simulink model "hil_tuning"  (R2018a)
settings: Solver=FixedStepAuto  StartTime=0.0  StopTime=inf  FixedStep=0.001  RelTol=1e-3  EnableMultiTasking=on
undefined symbols (not defined in the file or in its folder): d
libraries: simulink x12, xpcrtudplib x3, xpcseriallib x2
settings Model: SimulationMode=external  Creator=KLETech  LastModifiedBy=KLETech
settings SolverCC: ConcurrentTasks=on  AutoInsertRateTranBlk=on
settings DataIOCC: SaveFormat=StructureWithTime
settings OptimizationCC: BlockReduction=off  OptimizeBlockIOStorage=off  BufferReuse=off  GlobalBufferReuse=off  ExpressionFolding=off  LocalBlockOutputs=off  OptimizeDataStoreBuffers=off  BusAssignmentInplaceUpdate=off
settings HardwareCC: ProdBitPerPointer=32  ProdBitPerSizeT=32  ProdBitPerPtrDiffT=32  ProdLargestAtomicFloat=None  ProdWordSize=32  ProdLongLongMode=on  ProdHWDeviceType=Generic->32-bit x86 compatible
settings RTWCC: SystemTargetFile=slrt.tlc  TemplateMakefile=slrt_default_tmf  Description=Simulink Real-Time  CodeExecutionProfiling=on  RTWCompilerOptimization=on
settings SimulinkRealTimeCC: SupportVariableSizeSignals=on  RL32LogTETModifier=off  xPCConcurrentTasks=on

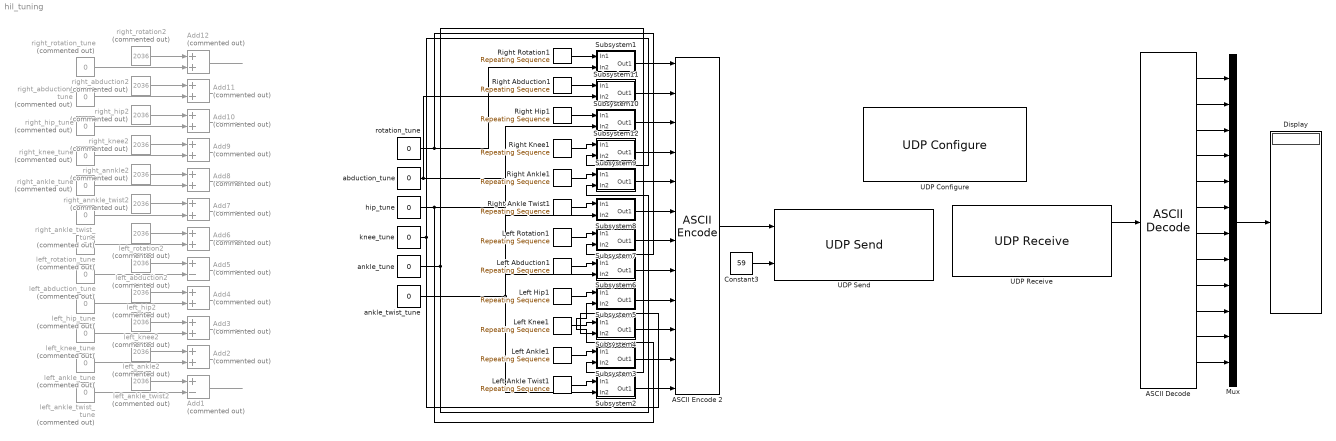
== system hil_tuning ==
  "ASCII Decode " : xpcseriallib/ASCII Decode   format=%d,%d,%d,%d,%d,%d,%d,%d,%d,%d,%d,%d  nvars=12  vartypes={ 'uint32' }
      settings: SourceProductName=Simulink Real-Time  SourceProductBaseCode=XP
  ASCII Encode 2 : xpcseriallib/ASCII Encode   format=%d,%d,%d,%d,%d,%d,%d,%d,%d,%d,%d,%d  nvars=12  maxlength=128  vartypes={ 'uint32' }
      settings: SourceProductName=Simulink Real-Time  SourceProductBaseCode=XP
  Add1 : Sum  Commented=on  Inputs=+-  OutDataTypeStr=uint32
  Add{2..4,6..12} (10 alike) : Sum  Commented=on  OutDataTypeStr=uint32
  Add5 : Sum  Commented=on  Inputs=+-  OutDataTypeStr=uint32
  Constant3 : Constant  Value=59
  Display : Display
  Left Abduction1 : simulink/Sources/Repeating Sequence  rep_seq_t=time  rep_seq_y=left_abduction
  Left Ankle Twist1 : simulink/Sources/Repeating Sequence  rep_seq_t=time  rep_seq_y=left_knee_twist
  Left Ankle1 : simulink/Sources/Repeating Sequence  rep_seq_t=time  rep_seq_y=left_ankle
  Left Hip1 : simulink/Sources/Repeating Sequence  rep_seq_t=time  rep_seq_y=left_hip
  Left Knee1 : simulink/Sources/Repeating Sequence  rep_seq_t=time  rep_seq_y=left_knee
  Left Rotation1 : simulink/Sources/Repeating Sequence  rep_seq_t=time  rep_seq_y=left_rotation
  Mux : Mux  Inputs=12
  Right Abduction1 : simulink/Sources/Repeating Sequence  rep_seq_t=time  rep_seq_y=right_abduction
  Right Ankle Twist1 : simulink/Sources/Repeating Sequence  rep_seq_t=time  rep_seq_y=right_knee_twist
  Right Ankle1 : simulink/Sources/Repeating Sequence  rep_seq_t=time  rep_seq_y=right_ankle
  Right Hip1 : simulink/Sources/Repeating Sequence  rep_seq_t=time  rep_seq_y=right_hip
  Right Knee1 : simulink/Sources/Repeating Sequence  rep_seq_t=time  rep_seq_y=right_knee
  Right Rotation1 : simulink/Sources/Repeating Sequence  rep_seq_t=time  rep_seq_y=right_rotation
  Subsystem1 : Subsystem
  Subsystem10 : Subsystem
  Subsystem11 : Subsystem
  Subsystem12 : Subsystem
  Subsystem2 : Subsystem
  Subsystem3 : Subsystem
  Subsystem4 : Subsystem
  Subsystem5 : Subsystem
  Subsystem6 : Subsystem
  Subsystem7 : Subsystem
  Subsystem8 : Subsystem
  Subsystem9 : Subsystem
  UDP Configure : xpcrtudplib/UDP Configure  Priority=-1  IpAddress=192.168.7.3  SubnetMask=255.0.0.0  Gateway=0.0.0.0  PciBus=[2]  PciSlot=[0]  PciFunction=0  ID=1  tune=0  enableMulticast=on  MulticastIpAddress={}  MulticastMask={}
      settings: SourceProductName=Simulink Real-Time  SourceProductBaseCode=XP
  UDP Receive : xpcrtudplib/UDP Receive  ipAddressVal=192.168.7.3  localPort=1234  rcvWidth=128  rcvFmAny=off  fmAddress=192.168.2.101  rcvMulticast=off  multicastAddress=[]  maxUDPQueue=8  sampleTime=-1
      settings: SourceProductName=Simulink Real-Time
  UDP Send : xpcrtudplib/UDP Send  ipAddressVal=192.168.7.3  localPort=25001  toAddress=192.168.2.101  toPort=8001  sampleTime=-1
      settings: SourceProductName=Simulink Real-Time  SourceProductBaseCode=XP
  abduction_tune : Constant  Value=0
  ankle_tune : Constant  Value=0
  ankle_twist_tune : Constant  Value=0
  hip_tune : Constant  Value=0
  knee_tune : Constant  Value=0
  "left_abduction2 " : Constant  Commented=on  Value=2036  OutDataTypeStr=uint32
  left_abduction_tune : Constant  Commented=on  Value=0  OutDataTypeStr=int32
  left_ankle2 : Constant  Commented=on  Value=2036  OutDataTypeStr=uint32
  left_ankle_tune : Constant  Commented=on  Value=0  OutDataTypeStr=int32
  "left_ankle_twist2 " : Constant  Commented=on  Value=2036  OutDataTypeStr=uint32
  left_ankle_twist_tune : Constant  Commented=on  Value=0  OutDataTypeStr=int32
  "left_hip2 " : Constant  Commented=on  Value=2036  OutDataTypeStr=uint32
  left_hip_tune : Constant  Commented=on  Value=0  OutDataTypeStr=int32
  left_knee2 : Constant  Commented=on  Value=2036  OutDataTypeStr=uint32
  left_knee_tune : Constant  Commented=on  Value=0  OutDataTypeStr=int32
  "left_rotation2 " : Constant  Commented=on  Value=2036  OutDataTypeStr=uint32
  left_rotation_tune : Constant  Commented=on  Value=0  OutDataTypeStr=int32
  "right_abduction2 " : Constant  Commented=on  Value=2036  OutDataTypeStr=uint32
  right_abduction_tune : Constant  Commented=on  Value=0  OutDataTypeStr=int32
  right_ankle_tune : Constant  Commented=on  Value=0  OutDataTypeStr=int32
  right_ankle_twist_tune : Constant  Commented=on  Value=0  OutDataTypeStr=int32
  right_annkle2 : Constant  Commented=on  Value=2036  OutDataTypeStr=uint32
  "right_annkle_twist2 " : Constant  Commented=on  Value=2036  OutDataTypeStr=uint32
  "right_hip2 " : Constant  Commented=on  Value=2036  OutDataTypeStr=uint32
  right_hip_tune : Constant  Commented=on  Value=0  OutDataTypeStr=int32
  right_knee2 : Constant  Commented=on  Value=2036  OutDataTypeStr=uint32
  right_knee_tune : Constant  Commented=on  Value=0  OutDataTypeStr=int32
  right_rotation2 : Constant  Commented=on  Value=2036  OutDataTypeStr=uint32
  right_rotation_tune : Constant  Commented=on  Value=0  OutDataTypeStr=int32
  rotation_tune : Constant  Value=0
  wires:
  ASCII Encode 2/1 -> UDP Send/1
  Constant3/1 -> UDP Send/2
  UDP Receive/1 -> "ASCII Decode "/1
  "ASCII Decode "/1 -> Mux/1
  "ASCII Decode "/2 -> Mux/2
  "ASCII Decode "/3 -> Mux/3
  "ASCII Decode "/4 -> Mux/4
  "ASCII Decode "/5 -> Mux/5
  "ASCII Decode "/6 -> Mux/6
  "ASCII Decode "/7 -> Mux/7
  "ASCII Decode "/8 -> Mux/8
  "ASCII Decode "/9 -> Mux/9
  "ASCII Decode "/10 -> Mux/10
  "ASCII Decode "/11 -> Mux/11
  "ASCII Decode "/12 -> Mux/12
  Mux/1 -> Display/1
  Subsystem7/1(Out1) -> ASCII Encode 2/7
  Subsystem1/1(Out1) -> ASCII Encode 2/1
  Subsystem10/1(Out1) -> ASCII Encode 2/3
  Subsystem12/1(Out1) -> ASCII Encode 2/4
  Subsystem9/1(Out1) -> ASCII Encode 2/5
  Subsystem5/1(Out1) -> ASCII Encode 2/9
  Subsystem3/1(Out1) -> ASCII Encode 2/11
  Subsystem11/1(Out1) -> ASCII Encode 2/2
  Subsystem4/1(Out1) -> ASCII Encode 2/10
  Right Abduction1/1 -> Subsystem11/1(In1)
  Right Rotation1/1 -> Subsystem1/1(In1)
  Left Rotation1/1 -> Subsystem7/1(In1)
  Subsystem8/1(Out1) -> ASCII Encode 2/6
  Subsystem6/1(Out1) -> ASCII Encode 2/8
  Subsystem2/1(Out1) -> ASCII Encode 2/12
  Left Ankle Twist1/1 -> Subsystem2/1(In1)
  Left Ankle1/1 -> Subsystem3/1(In1)
  Right Ankle Twist1/1 -> Subsystem8/1(In1)
  Left Hip1/1 -> Subsystem5/1(In1)
  Left Knee1/1 -> Subsystem4/1(In1)
  Right Ankle1/1 -> Subsystem9/1(In1)
  Right Knee1/1 -> Subsystem12/1(In1)
  Right Hip1/1 -> Subsystem10/1(In1)
  Left Abduction1/1 -> Subsystem6/1(In1)
  "left_ankle_twist2 "/1 -> Add1/1
  "right_abduction2 "/1 -> Add11/1
  "right_hip2 "/1 -> Add10/1
  left_knee2/1 -> Add3/1
  right_knee2/1 -> Add9/1
  "left_abduction2 "/1 -> Add5/1
  left_ankle2/1 -> Add2/1
  "left_rotation2 "/1 -> Add6/1
  right_rotation2/1 -> Add12/1
  left_ankle_tune/1 -> Add2/2
  right_knee_tune/1 -> Add9/2
  left_rotation_tune/1 -> Add6/2
  right_hip_tune/1 -> Add10/2
  left_abduction_tune/1 -> Add5/2
  right_abduction_tune/1 -> Add11/2
  right_ankle_tune/1 -> Add8/2
  left_knee_tune/1 -> Add3/2
  right_ankle_twist_tune/1 -> Add7/2
  left_hip_tune/1 -> Add4/2
  right_rotation_tune/1 -> Add12/2
  Add6/1 -> ?
  right_annkle2/1 -> Add8/1
  Add10/1 -> ?
  Add12/1 -> ?
  "left_hip2 "/1 -> Add4/1
  Add1/1 -> ?
  Add4/1 -> ?
  Add2/1 -> ?
  Add8/1 -> ?
  Add3/1 -> ?
  "right_annkle_twist2 "/1 -> Add7/1
  Add11/1 -> ?
  Add9/1 -> ?
  Add7/1 -> ?
  Add5/1 -> ?
  left_ankle_twist_tune/1 -> Add1/2
  ankle_twist_tune/1 -> Subsystem8/2(In2), Subsystem2/2(In2)
  ankle_tune/1 -> Subsystem9/2(In2), Subsystem3/2(In2)
  knee_tune/1 -> Subsystem12/2(In2), Subsystem4/2(In2)
  hip_tune/1 -> Subsystem10/2(In2), Subsystem5/2(In2)
  abduction_tune/1 -> Subsystem11/2(In2), Subsystem6/2(In2)
  rotation_tune/1 -> Subsystem7/2(In2), Subsystem1/2(In2)

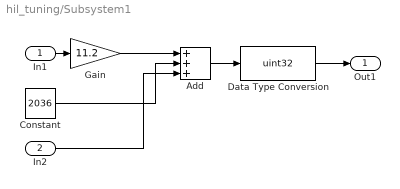
== system hil_tuning/Subsystem1 ==
  In1 : Inport
  In2 : Inport  Port=2
  Add : Sum  Inputs=+++
  Constant : Constant  Value=2036
  Data Type Conversion : DataTypeConversion  OutDataTypeStr=uint32
  Gain : Gain  Gain=11.2
  Out1 : Outport
  wires:
  Add/1 -> Data Type Conversion/1
  Gain/1 -> Add/1
  Constant/1 -> Add/2
  In1/1 -> Gain/1
  Data Type Conversion/1 -> Out1/1
  In2/1 -> Add/3

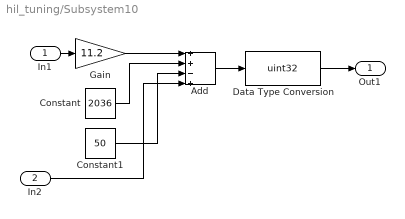
== system hil_tuning/Subsystem10 ==
  In1 : Inport
  In2 : Inport  Port=2
  Add : Sum  Inputs=++-+
  Constant : Constant  Value=2036
  Constant1 : Constant  Value=50
  Data Type Conversion : DataTypeConversion  OutDataTypeStr=uint32
  Gain : Gain  Gain=11.2
  Out1 : Outport
  wires:
  Add/1 -> Data Type Conversion/1
  Gain/1 -> Add/1
  Constant/1 -> Add/2
  In1/1 -> Gain/1
  Data Type Conversion/1 -> Out1/1
  Constant1/1 -> Add/3
  In2/1 -> Add/4

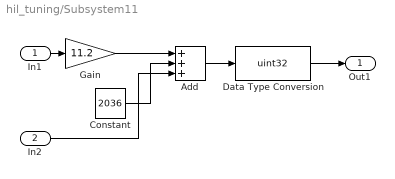
== system hil_tuning/Subsystem11 ==
  In1 : Inport
  In2 : Inport  Port=2
  Add : Sum  Inputs=+++
  Constant : Constant  Value=2036
  Data Type Conversion : DataTypeConversion  OutDataTypeStr=uint32
  Gain : Gain  Gain=11.2
  Out1 : Outport
  wires:
  Add/1 -> Data Type Conversion/1
  Gain/1 -> Add/1
  Constant/1 -> Add/2
  In1/1 -> Gain/1
  Data Type Conversion/1 -> Out1/1
  In2/1 -> Add/3

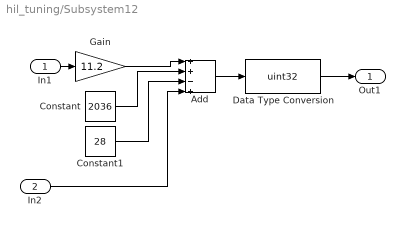
== system hil_tuning/Subsystem12 ==
  In1 : Inport
  In2 : Inport  Port=2
  Add : Sum  Inputs=++-+
  Constant : Constant  Value=2036
  Constant1 : Constant  Value=28
  Data Type Conversion : DataTypeConversion  OutDataTypeStr=uint32
  Gain : Gain  Gain=11.2
  Out1 : Outport
  wires:
  Add/1 -> Data Type Conversion/1
  Gain/1 -> Add/1
  Constant/1 -> Add/2
  In1/1 -> Gain/1
  Data Type Conversion/1 -> Out1/1
  Constant1/1 -> Add/3
  In2/1 -> Add/4

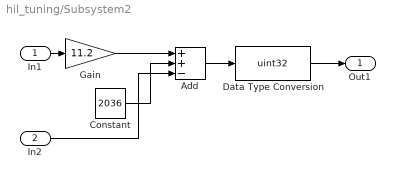
== system hil_tuning/Subsystem2 ==
  In1 : Inport
  In2 : Inport  Port=2
  Add : Sum  Inputs=++-
  Constant : Constant  Value=2036
  Data Type Conversion : DataTypeConversion  OutDataTypeStr=uint32
  Gain : Gain  Gain=11.2
  Out1 : Outport
  wires:
  Add/1 -> Data Type Conversion/1
  Gain/1 -> Add/1
  Constant/1 -> Add/2
  In1/1 -> Gain/1
  Data Type Conversion/1 -> Out1/1
  In2/1 -> Add/3

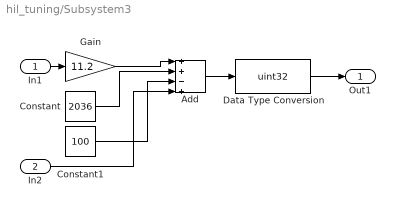
== system hil_tuning/Subsystem3 ==
  In1 : Inport
  In2 : Inport  Port=2
  Add : Sum  Inputs=++-+
  Constant : Constant  Value=2036
  Constant1 : Constant  Value=100
  Data Type Conversion : DataTypeConversion  OutDataTypeStr=uint32
  Gain : Gain  Gain=11.2
  Out1 : Outport
  wires:
  Add/1 -> Data Type Conversion/1
  Gain/1 -> Add/1
  Constant/1 -> Add/2
  In1/1 -> Gain/1
  Data Type Conversion/1 -> Out1/1
  Constant1/1 -> Add/3
  In2/1 -> Add/4

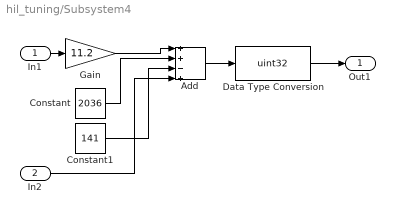
== system hil_tuning/Subsystem4 ==
  In1 : Inport
  In2 : Inport  Port=2
  Add : Sum  Inputs=++-+
  Constant : Constant  Value=2036
  Constant1 : Constant  Value=141
  Data Type Conversion : DataTypeConversion  OutDataTypeStr=uint32
  Gain : Gain  Gain=11.2
  Out1 : Outport
  wires:
  Add/1 -> Data Type Conversion/1
  Gain/1 -> Add/1
  Constant/1 -> Add/2
  In1/1 -> Gain/1
  Data Type Conversion/1 -> Out1/1
  Constant1/1 -> Add/3
  In2/1 -> Add/4

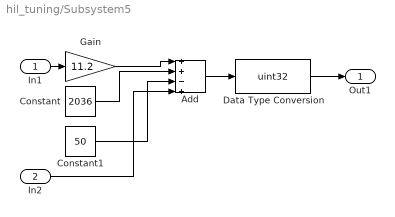
== system hil_tuning/Subsystem5 ==
  In1 : Inport
  In2 : Inport  Port=2
  Add : Sum  Inputs=++-+
  Constant : Constant  Value=2036
  Constant1 : Constant  Value=50
  Data Type Conversion : DataTypeConversion  OutDataTypeStr=uint32
  Gain : Gain  Gain=11.2
  Out1 : Outport
  wires:
  Add/1 -> Data Type Conversion/1
  Gain/1 -> Add/1
  Constant/1 -> Add/2
  In1/1 -> Gain/1
  Data Type Conversion/1 -> Out1/1
  Constant1/1 -> Add/3
  In2/1 -> Add/4

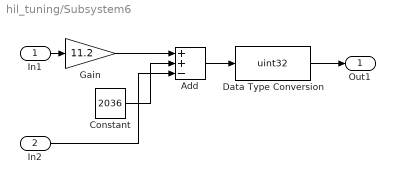
== system hil_tuning/Subsystem6 ==
  In1 : Inport
  In2 : Inport  Port=2
  Add : Sum  Inputs=++-
  Constant : Constant  Value=2036
  Data Type Conversion : DataTypeConversion  OutDataTypeStr=uint32
  Gain : Gain  Gain=11.2
  Out1 : Outport
  wires:
  Add/1 -> Data Type Conversion/1
  Gain/1 -> Add/1
  Constant/1 -> Add/2
  In1/1 -> Gain/1
  Data Type Conversion/1 -> Out1/1
  In2/1 -> Add/3

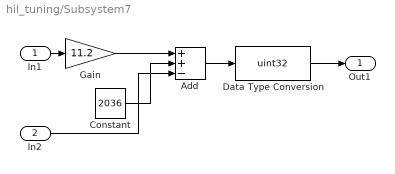
== system hil_tuning/Subsystem7 ==
  In1 : Inport
  In2 : Inport  Port=2
  Add : Sum  Inputs=++-
  Constant : Constant  Value=2036
  Data Type Conversion : DataTypeConversion  OutDataTypeStr=uint32
  Gain : Gain  Gain=11.2
  Out1 : Outport
  wires:
  Add/1 -> Data Type Conversion/1
  Gain/1 -> Add/1
  Constant/1 -> Add/2
  In1/1 -> Gain/1
  Data Type Conversion/1 -> Out1/1
  In2/1 -> Add/3

== system hil_tuning/Subsystem8 ==
  In1 : Inport
  In2 : Inport  Port=2
  Add : Sum  Inputs=+++
  Constant : Constant  Value=2036
  Data Type Conversion : DataTypeConversion  OutDataTypeStr=uint32
  Gain : Gain  Gain=11.2
  Out1 : Outport
  wires:
  Add/1 -> Data Type Conversion/1
  Gain/1 -> Add/1
  Constant/1 -> Add/2
  In1/1 -> Gain/1
  Data Type Conversion/1 -> Out1/1
  In2/1 -> Add/3

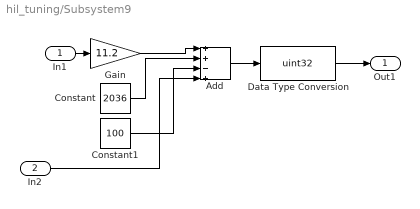
== system hil_tuning/Subsystem9 ==
  In1 : Inport
  In2 : Inport  Port=2
  Add : Sum  Inputs=++-+
  Constant : Constant  Value=2036
  Constant1 : Constant  Value=100
  Data Type Conversion : DataTypeConversion  OutDataTypeStr=uint32
  Gain : Gain  Gain=11.2
  Out1 : Outport
  wires:
  Add/1 -> Data Type Conversion/1
  Gain/1 -> Add/1
  Constant/1 -> Add/2
  In1/1 -> Gain/1
  Data Type Conversion/1 -> Out1/1
  Constant1/1 -> Add/3
  In2/1 -> Add/4
